simulink model "PathTrackingSensorModel"  (R2026b)
settings: Solver=ode4  StopTime=10  FixedStep=0.01
settings Model: DataDictionary=VehicleData.sldd  Creator=Xu Dingyi  LastModifiedBy=29358

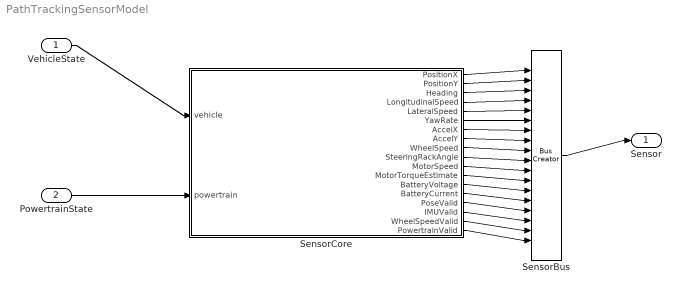
== system PathTrackingSensorModel ==
  VehicleState : Inport  OutDataTypeStr=Bus: VehicleStateBus
  PowertrainState : Inport  Port=2  OutDataTypeStr=Bus: PowertrainStateBus
  SensorBus : BusCreator  Inputs=18  OutDataTypeStr=Bus: SensorBus
  SensorCore : MATLAB Function  TreatAsAtomicUnit=on
  Sensor : Outport  OutDataTypeStr=Bus: SensorBus
  wires:
  VehicleState/1 -> SensorCore/1(vehicle)
  PowertrainState/1 -> SensorCore/2(powertrain)
  SensorCore/1(PositionX) -> SensorBus/1
  SensorCore/2(PositionY) -> SensorBus/2
  SensorCore/3(Heading) -> SensorBus/3
  SensorCore/4(LongitudinalSpeed) -> SensorBus/4
  SensorCore/5(LateralSpeed) -> SensorBus/5
  SensorCore/6(YawRate) -> SensorBus/6
  SensorCore/7(AccelX) -> SensorBus/7
  SensorCore/8(AccelY) -> SensorBus/8
  SensorCore/9(WheelSpeed) -> SensorBus/9
  SensorCore/10(SteeringRackAngle) -> SensorBus/10
  SensorCore/11(MotorSpeed) -> SensorBus/11
  SensorCore/12(MotorTorqueEstimate) -> SensorBus/12
  SensorCore/13(BatteryVoltage) -> SensorBus/13
  SensorCore/14(BatteryCurrent) -> SensorBus/14
  SensorCore/15(PoseValid) -> SensorBus/15
  SensorCore/16(IMUValid) -> SensorBus/16
  SensorCore/17(WheelSpeedValid) -> SensorBus/17
  SensorCore/18(PowertrainValid) -> SensorBus/18
  SensorBus/1 -> Sensor/1

== matlab function PathTrackingSensorModel/SensorCore ==
  data: vehicle input; PositionX output; powertrain input; PositionY output; Heading output; LongitudinalSpeed output; LateralSpeed output; YawRate output; AccelX output; AccelY output; WheelSpeed output; SteeringRackAngle output; MotorSpeed output; MotorTorqueEstimate output; BatteryVoltage output; BatteryCurrent output; PoseValid output; IMUValid output; WheelSpeedValid output; PowertrainValid output
function [PositionX, PositionY, Heading, LongitudinalSpeed, LateralSpeed, ...
    YawRate, AccelX, AccelY, WheelSpeed, SteeringRackAngle, MotorSpeed, ...
    MotorTorqueEstimate, BatteryVoltage, BatteryCurrent, PoseValid, ...
    IMUValid, WheelSpeedValid, PowertrainValid] = ...
    fcn(vehicle, powertrain)
%FSAEPathTrackingSENSORCORE Truth-derived sensor emulation for PathTracking MIL.
%   No tire force or friction truth is exposed.  Noise, latency and an
%   estimator are intentionally deferred to the deployment milestone.

PositionX = vehicle.X;
PositionY = vehicle.Y;
Heading = vehicle.Psi;
LongitudinalSpeed = vehicle.Ux;
LateralSpeed = vehicle.Uy;
YawRate = vehicle.YawRate;
AccelX = vehicle.Ax;
AccelY = vehicle.Ay;
WheelSpeed = vehicle.WheelSpeed;
SteeringRackAngle = mean(vehicle.WheelSteerAngle(1:2));
MotorSpeed = powertrain.MotorSpeed;
MotorTorqueEstimate = powertrain.MotorTorqueActual;
BatteryVoltage = powertrain.BatteryVoltage;
BatteryCurrent = powertrain.BatteryCurrent;
PoseValid = true;
IMUValid = true;
WheelSpeedValid = true(4, 1);
PowertrainValid = true;
end
